simulink model "HWILSimulinkToGUITest"  (R2022b)
settings: Solver=VariableStepAuto  StartTime=0.0  StopTime=10.0  RelTol=1e-3
libraries: instrumentlib x3, vrlib x1
settings Model: Creator=jrsan  LastModifiedBy=jrsan
settings DebuggingCC: UnconnectedInputMsg=warning  UnconnectedOutputMsg=warning  UnconnectedLineMsg=warning
settings ModelReferenceCC: EnableRefExpFcnMdlSchedulingChecks=on
settings RTWCC: DLArmComputeVersion=19.05

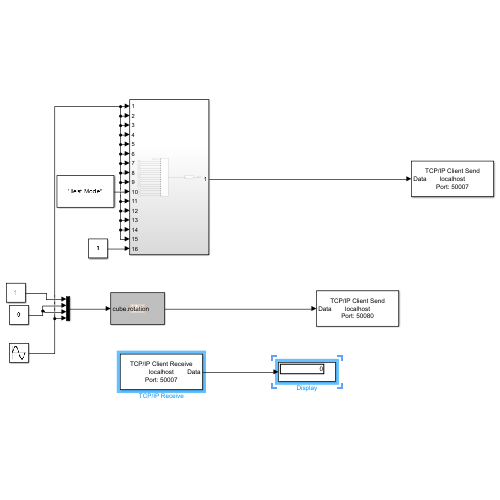
[thumbnail: Simulink's stored preview of the top-level diagram]
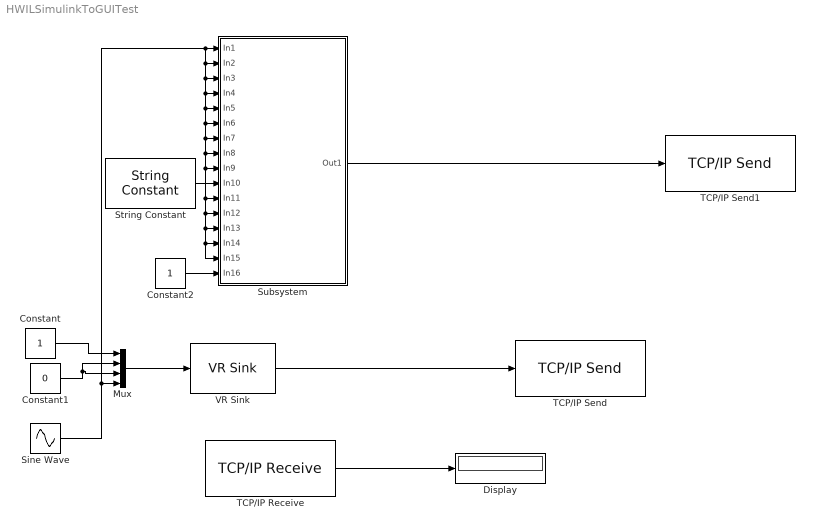
== system HWILSimulinkToGUITest ==
  Constant : Constant
  Constant1 : Constant  Value=0
  Constant2 : Constant
  Display : Display
  Mux : Mux
  Sine Wave : Sin  SampleTime=0
  String Constant : StringConstant  String="\"Test Mode\""
  Subsystem : Subsystem
  TCP/IP Receive : instrumentlib/TCP//IP Receive  Host=localhost  Port=50007  DataSize=[ 1, 1 ]  DataType=ASCII  ASCIIFormatting=%f  Terminator=LF  CustomTerminator=10  ByteOrder=big-endian  EnableBlockingMode=on  Timeout=10  SampleTime=0.01  SimulateUsing=Interpreted execution
  TCP/IP Send : instrumentlib/TCP//IP Send  Host=localhost  Port=50080  ByteOrder=big-endian  EnableBlockingMode=on  Timeout=10  TransferDelay=on  SimulateUsing=Interpreted execution
  TCP/IP Send1 : instrumentlib/TCP//IP Send  Host=localhost  Port=50007  ByteOrder=big-endian  EnableBlockingMode=on  Timeout=10  TransferDelay=on  SimulateUsing=Interpreted execution
  VR Sink : vrlib/VR Sink  InstantiateOnLoad=on  SampleTime=0.1  ViewEnable=on  RemoteChange=off  RemoteView=off  FieldsWritten=cube.rotation.4.1.1.double  WorldFileName=TestEnvironment.wrl  AutoView=on  VideoDimensions=[600 600]  AllowVariableSize=off  FigureProperties="{'Position', 'Name', 'Viewpoint', 'CameraBound', 'CameraDirection', 'CameraPosition', 'CameraUpVector', 'ZoomFactor', 'Antialiasing', 'Headlight', 'Lighting', 'NavPanel', 'Sound', 'StatusBar', 'Stereo3D', 'Stereo3DCameraOffset', 'Stereo3DHIT', 'ToolBar', 'Textures', 'Transparency', 'Triad', 'Wireframe', 'NavZones', 'NavMode', 'NavSpeed', 'CaptureFileFormat', 'CaptureFileName', 'Record2DCompressMethod', 'Record2DCompressQuality', 'Record2D', 'Record2DFileName', 'Record2DFPS'; [2.2900000000000000e+02   1.8300000000000000e+02   5.7600000000000000e+02   3.5000000000000000e+02], '', '_untitled_1', 'on', [0.0000000000000000e+00   0.0000000000000000e+00  -1.0000000000000000e+00], [0.0000000000000000e+00   0.0000000000000000e+00   0.0000000000000000e+00], [0.0000000000000000e+00   1.0000000000000000e+00   0.0000000000000000e+00], [1.0000000000000000e+00], 'off', 'on', 'on', 'halfbar', 'on', 'on', 'off', [1.0000000149011612e-01], [0.0000000000000000e+00], 'on', 'on', 'on', 'none', 'off', 'off', 'fly', 'normal', 'tif', '%f_anim_%n.tif', 'auto', [7.5000000000000000e+01], 'off', '%f_anim_%n.avi', 'auto'; [5.0000000000000000e+00   1.4139999999999998e+02   7.2000000000000000e+02   7.2000000000000000e+02], '', '_untitled_1', 'on', [2.9464090179904684e-01  -1.2782615481716345e-01  -9.4702017567299024e-01], [-1.7044157259176573e+00   4.3677417675225805e-01   2.4614770772074754e+00], [1.1013951458365309e-01   9.8895141815049903e-01  -9.9218848337364052e-02], [1.0000000000000000e+00], 'on', 'on', 'on', 'none', 'on', 'off', 'off', [1.0000000149011612e-01], [0.0000000000000000e+00], 'off', 'on', 'on', 'none', 'off', 'off', 'fly', 'normal', 'tif', '%f_anim_%n.tif', 'auto', [7.5000000000000000e+01], 'off', '***video***', 'auto'}"
  wires:
  Mux/1 -> VR Sink/1
  Constant/1 -> Mux/1
  Constant1/1 -> Mux/3, Mux/2
  Sine Wave/1 -> Subsystem/2(In2), Subsystem/15(In15), Subsystem/14(In14), Subsystem/13(In13), Subsystem/12(In12), Subsystem/11(In11), Subsystem/9(In9), Subsystem/8(In8), Subsystem/7(In7), Subsystem/6(In6), Subsystem/5(In5), Subsystem/4(In4), Subsystem/3(In3), Subsystem/1(In1), Mux/4
  TCP/IP Receive/1 -> Display/1
  Subsystem/1(Out1) -> TCP/IP Send1/1
  Constant2/1 -> Subsystem/16(In16)
  String Constant/1 -> Subsystem/10(In10)
  VR Sink/1 -> TCP/IP Send/1

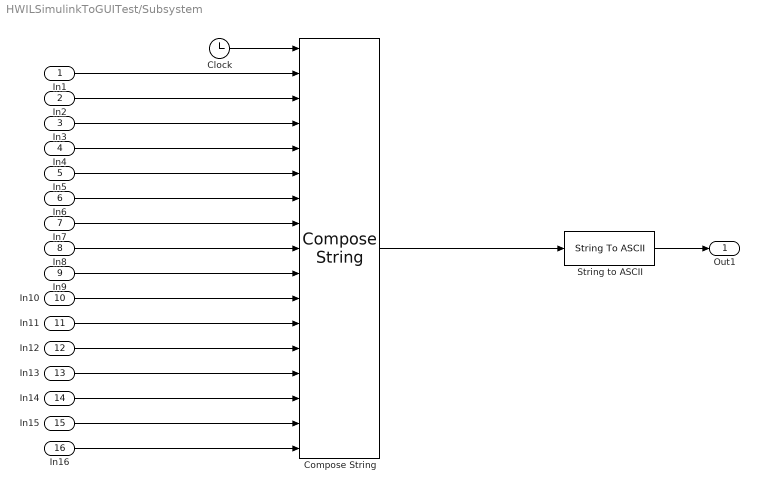
== system HWILSimulinkToGUITest/Subsystem ==
  In1 : Inport
  In2 : Inport  Port=2
  In3 : Inport  Port=3
  In4 : Inport  Port=4
  In5 : Inport  Port=5
  In6 : Inport  Port=6
  In7 : Inport  Port=7
  In8 : Inport  Port=8
  In9 : Inport  Port=9
  In10 : Inport  Port=10
  In11 : Inport  Port=11
  In12 : Inport  Port=12
  In13 : Inport  Port=13
  In14 : Inport  Port=14
  In15 : Inport  Port=15
  In16 : Inport  Port=16
  Clock : Clock
  Compose String : ComposeString  Format="\"%f,%f,%f,%f,%f,%f,%f,%f,%f,%f,%s,%f,%f,%f,%f,%f,%f,\""
  String to ASCII : StringToASCII  OutputVectorSize=256
  Out1 : Outport
  wires:
  In16/1 -> Compose String/17
  In15/1 -> Compose String/16
  In14/1 -> Compose String/15
  In13/1 -> Compose String/14
  In12/1 -> Compose String/13
  In11/1 -> Compose String/12
  In10/1 -> Compose String/11
  In9/1 -> Compose String/10
  In8/1 -> Compose String/9
  In7/1 -> Compose String/8
  In6/1 -> Compose String/7
  In5/1 -> Compose String/6
  In4/1 -> Compose String/5
  In3/1 -> Compose String/4
  In2/1 -> Compose String/3
  In1/1 -> Compose String/2
  Clock/1 -> Compose String/1
  Compose String/1 -> String to ASCII/1
  String to ASCII/1 -> Out1/1
